simulink library "Desaturation_Controller_lib"  (R2018b)
settings: Solver=VariableStepAuto  StartTime=0.0  StopTime=10.0  RelTol=1e-3
undefined symbols (not defined in the file or in its folder): fswParams
libraries: Div_by_0_protection x2, vrlib x1
settings Model: Creator=colem  LastModifiedBy=colem

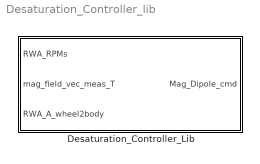
== system Desaturation_Controller_lib ==
  Desaturation_Controller_Lib : Subsystem

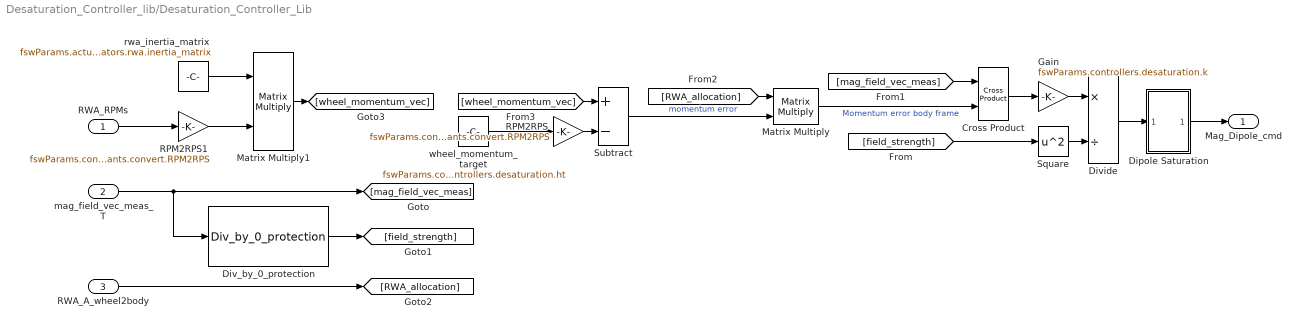
== system Desaturation_Controller_lib/Desaturation_Controller_Lib ==
  RWA_RPMs : Inport
  mag_field_vec_meas_T : Inport  Port=2
  RWA_A_wheel2body : Inport  Port=3
  Cross Product : vrlib/Utilities/Cross Product
      settings: SourceProductBaseCode=VR
  Dipole Saturation : Subsystem
  Div_by_0_protection : Div_by_0_protection/Div_by_0_protection  SystemSampleTime=-1
  Divide : Product  Inputs=*/
  Gain : Gain  Gain=fswParams.controllers.desaturation.k
  Matrix Multiply : Product  Multiplication=Matrix(*)
  Matrix Multiply1 : Product  Multiplication=Matrix(*)
  RPM2RPS : Gain  Gain=fswParams.constants.convert.RPM2RPS
  RPM2RPS1 : Gain  Gain=fswParams.constants.convert.RPM2RPS
  Square : Math  Operator=square  SaturateOnIntegerOverflow=on
  Subtract : Sum  Inputs=+-
  rwa_inertia_matrix : Constant  Value=fswParams.actuators.rwa.inertia_matrix  SampleTime=fswParams.sample_time_s
  wheel_momentum_target : Constant  Value=fswParams.controllers.desaturation.ht  SampleTime=fswParams.sample_time_s
  Mag_Dipole_cmd : Outport
  wires:
  [RWA_allocation] -> Matrix Multiply/1
  Matrix Multiply/1 -> Cross Product/2  "Momentum error body frame"
  Subtract/1 -> Matrix Multiply/2  "momentum error"
  Cross Product/1 -> Gain/1
  RWA_RPMs/1 -> RPM2RPS1/1
  Gain/1 -> Divide/1
  mag_field_vec_meas_T/1 -> Div_by_0_protection/1, [mag_field_vec_meas]
  [field_strength] -> Square/1
  Square/1 -> Divide/2
  [mag_field_vec_meas] -> Cross Product/1
  RWA_A_wheel2body/1 -> [RWA_allocation]
  rwa_inertia_matrix/1 -> Matrix Multiply1/1
  Matrix Multiply1/1 -> [wheel_momentum_vec]
  [wheel_momentum_vec] -> Subtract/1
  wheel_momentum_target/1 -> RPM2RPS/1
  Divide/1 -> Dipole Saturation/1(In1)
  Div_by_0_protection/1 -> [field_strength]
  RPM2RPS/1 -> Subtract/2
  RPM2RPS1/1 -> Matrix Multiply1/2
  Dipole Saturation/1(Out1) -> Mag_Dipole_cmd/1

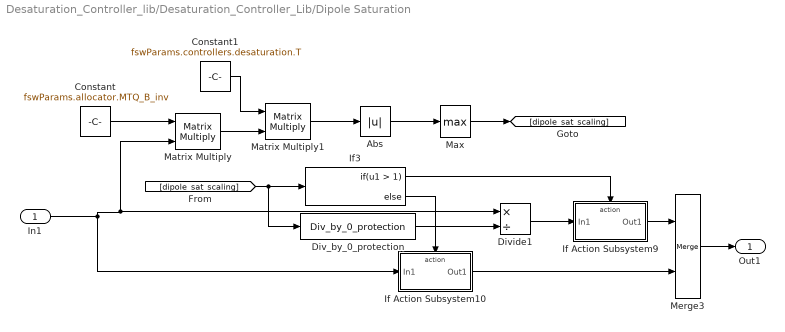
== system Desaturation_Controller_lib/Desaturation_Controller_Lib/Dipole Saturation ==
  In1 : Inport
  Abs : Abs
  Constant : Constant  Value=fswParams.allocator.MTQ_B_inv  SampleTime=fswParams.sample_time_s
  Constant1 : Constant  Value=fswParams.controllers.desaturation.T  SampleTime=fswParams.sample_time_s
  Div_by_0_protection : Div_by_0_protection/Div_by_0_protection  SystemSampleTime=-1
  Divide1 : Product  Inputs=*/
  If Action Subsystem10 : Subsystem  TreatAsAtomicUnit=on
  If Action Subsystem9 : Subsystem  TreatAsAtomicUnit=on
  If3 : If  IfExpression=u1 > 1
  Matrix Multiply : Product  Multiplication=Matrix(*)
  Matrix Multiply1 : Product  Multiplication=Matrix(*)
  Max : MinMax  Function=max
  Merge3 : Merge
  Out1 : Outport
  wires:
  If Action Subsystem9/1(Out1) -> Merge3/1
  If3/1 -> If Action Subsystem9/Action
  If3/2 -> If Action Subsystem10/Action
  If Action Subsystem10/1(Out1) -> Merge3/2
  Merge3/1 -> Out1/1
  Divide1/1 -> If Action Subsystem9/1(In1)
  Constant/1 -> Matrix Multiply/1
  In1/1 -> Matrix Multiply/2, Divide1/1, If Action Subsystem10/1(In1)
  Matrix Multiply/1 -> Matrix Multiply1/2
  Constant1/1 -> Matrix Multiply1/1
  Matrix Multiply1/1 -> Abs/1
  Abs/1 -> Max/1
  [dipole_sat_scaling] -> Div_by_0_protection/1, If3/1
  Max/1 -> [dipole_sat_scaling]
  Div_by_0_protection/1 -> Divide1/2

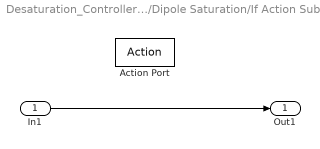
== system Desaturation_Controller_lib/Desaturation_Controller_Lib/Dipole Saturation/If Action Subsystem10 ==
  In1 : Inport
  Action Port : ActionPort
  Out1 : Outport
  wires:
  In1/1 -> Out1/1

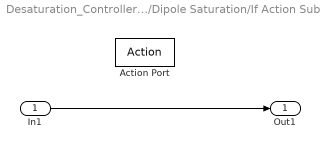
== system Desaturation_Controller_lib/Desaturation_Controller_Lib/Dipole Saturation/If Action Subsystem9 ==
  In1 : Inport
  Action Port : ActionPort
  Out1 : Outport
  wires:
  In1/1 -> Out1/1
